simulink model "Supplementary"  (R2021a)
(part 22 of 44)

  | 59.9400000000000	0.0230096000000000	0	0.251530791000000	0.179781140000000	-0.315026171000000	-0.0424638370000000	0	0.0447050030000000	0.252430607000000	0.117599632000000	-0.0562562650000000	0	-0.250118815000000	0.495220037000000	0.448104106000000	0.0380873640000000	0	0.457102020000000	-0.0355396720000000	0.0629174220000000	0.0269596900000000	0	0.0225587780000000	-0.198933159000000	-0.173880731000000	0.0329760380000000	0	-0.0120823110000000	-0.612381407000000	-0.0657713680000000
  | 59.9500000000000	0.0225821490000000	0	0.251965335000000	0.182330207000000	-0.313827770000000	-0.0430235900000000	0	0.0421946840000000	0.257386793000000	0.122104378000000	-0.0556942900000000	0	-0.251945003000000	0.496017229000000	0.452844988000000	0.0383586100000000	0	0.457327004000000	-0.0375596220000000	0.0611753260000000	0.0272837990000000	0	0.0224268220000000	-0.204964025000000	-0.174486467000000	0.0318457760000000	0	-0.0143088790000000	-0.593791789000000	-0.0553758650000000
  | 59.9600000000000	0.0221491290000000	0	0.252374684000000	0.184928876000000	-0.312584084000000	-0.0435777230000000	0	0.0396661030000000	0.262350951000000	0.126656532000000	-0.0551323150000000	0	-0.253771190000000	0.496814420000000	0.457585870000000	0.0386330400000000	0	0.457550556000000	-0.0396389520000000	0.0594276930000000	0.0275966060000000	0	0.0222726010000000	-0.210808995000000	-0.174988248000000	0.0307155150000000	0	-0.0165354480000000	-0.575202171000000	-0.0449803630000000
  | 59.9700000000000	0.0217105950000000	0	0.252758657000000	0.187577226000000	-0.311294639000000	-0.0441262360000000	0	0.0371192600000000	0.267323082000000	0.131256095000000	-0.0545703400000000	0	-0.255597377000000	0.497611611000000	0.462326751000000	0.0389105420000000	0	0.457772456000000	-0.0417758020000000	0.0576755610000000	0.0278981090000000	0	0.0220961140000000	-0.216468068000000	-0.175386074000000	0.0295852530000000	0	-0.0187620170000000	-0.556612554000000	-0.0345848600000000
  | 59.9800000000000	0.0212666040000000	0	0.253117069000000	0.190275337000000	-0.309958962000000	-0.0446691290000000	0	0.0345541550000000	0.272303184000000	0.135903067000000	-0.0540083650000000	0	-0.257423565000000	0.498408802000000	0.467067633000000	0.0391910020000000	0	0.457992479000000	-0.0439683140000000	0.0559199710000000	0.0281883110000000	0	0.0218973610000000	-0.221941246000000	-0.175679945000000	0.0284549920000000	0	-0.0209885860000000	-0.538022936000000	-0.0241893580000000
  | 59.9900000000000	0.0208172120000000	0	0.253449740000000	0.193023290000000	-0.308576578000000	-0.0452064030000000	0	0.0319707890000000	0.277291258000000	0.140597448000000	-0.0534388670000000	0	-0.259237508000000	0.499147350000000	0.471723171000000	0.0394743080000000	0	0.458210403000000	-0.0462146270000000	0.0541619620000000	0.0284672090000000	0	0.0216763420000000	-0.227228527000000	-0.175869861000000	0.0272789170000000	0	-0.0232242500000000	-0.519210865000000	-0.0136702450000000
  | 60	0.0203624760000000	0	0.253756485000000	0.195821163000000	-0.307147013000000	-0.0457379070000000	0	0.0293694050000000	0.282286131000000	0.145337530000000	-0.0528242280000000	0	-0.260977987000000	0.499534036000000	0.475866645000000	0.0397603470000000	0	0.458426005000000	-0.0485128840000000	0.0524025740000000	0.0287338890000000	0	0.0214328760000000	-0.232325463000000	-0.175953350000000	0.0258279680000000	0	-0.0255144850000000	-0.499064078000000	-0.00240947200000000]
StopFcn:
  | clc
  | close all
  | 
  | T = Time.Data(:);
  | 
  | 
  | LeftThighF = LThighF.Data(:,:);
  | LeftThighT = LThighT.Data(:,:);
  | LeftThighS = LThighS.Data(:,:);
  | LeftKnee   = LKnee.Data(:,:);
  | LeftAnkle  = LAnkle.Data(:,:);
  | 
  | RightThighF = RThighF.Data(:,:);
  | RightThighT = RThighT.Data(:,:);
  | RightThighS = RThighS.Data(:,:);
  | RightKnee   = RKnee.Data(:,:);
  | RightAnkle  = RAnkle.Data(:,:);
  | 
  | 
  | LeftThighFtorque = LThighFtorque.Data(:);
  | LeftThighTtorque = LThighTtorque.Data(:);
  | LeftThighStorque = LThighStorque.Data(:);
  | LeftKneetorque   = LKneetorque.Data(:);
  | LeftAnkletorque  = LAnkletorque.Data(:);
  | 
  | RightThighFtorque = RThighFtorque.Data(:);
  | RightThighTtorque = RThighTtorque.Data(:);
  | RightThighStorque = RThighStorque.Data(:);
  | RightKneetorque   = RKneetorque.Data(:);
  | RightAnkletorque  = RAnkletorque.Data(:);
  | 
  | 
  | figure
  | subplot(4,2,2)
  | plot(T,RightThighF(:,1),'g',T,RightThighF(:,2),'b',T,RightThighF(:,3),'--m' ,'LineWidth',3)
  | legend({'\theta_{Ref}','\theta_{Simscape}','\theta_{Simulink}'}, 'Location','northeast', 'FontSize',10,'FontName', 'Times New Roman', 'FontWeight', 'bold')
  | xlabel('Time (Sec)', 'FontSize',10,'FontName', 'Times New Roman', 'FontWeight', 'bold' )
  | ylabel('Position (Degree)', 'FontSize',10,'FontName', 'Times New Roman', 'FontWeight', 'bold' )
  | title('Right Frontal Hip Position', 'FontSize',10,'FontName', 'Times New Roman' , 'FontWeight', 'bold')
  | ax = gca;
  | ax.FontSize = 10;
  | ax.FontName = 'Times New Roman';
  | ax.FontWeight = 'bold';
  | grid on
  | 
  | 
  | 
  | subplot(4,2,4)
  | plot(T,RightThighS(:,1),'g',T,RightThighS(:,2),'b',T,RightThighS(:,3),'--m' ,'LineWidth',3)
  | legend({'\theta_{Ref}','\theta_{Simscape}','\theta_{Simulink}'}, 'Location','northeast', 'FontSize',10,'FontName', 'Times New Roman', 'FontWeight', 'bold')
  | xlabel('Time (Sec)', 'FontSize',10,'FontName', 'Times New Roman', 'FontWeight', 'bold' )
  | ylabel('Position (Degree)', 'FontSize',10,'FontName', 'Times New Roman', 'FontWeight', 'bold' )
  | title('Right Saggital Hip Position', 'FontSize',10,'FontName', 'Times New Roman' , 'FontWeight', 'bold')
  | ax = gca;
  | ax.FontSize = 10;
  | ax.FontName = 'Times New Roman';
  | ax.FontWeight = 'bold';
  | grid on
  | 
  | 
  | 
  | subplot(4,2,6)
  | plot(T,RightKnee(:,1),'g',T,RightKnee(:,2),'b',T,RightKnee(:,3),'--m' ,'LineWidth',3)
  | legend({'\theta_{Ref}','\theta_{Simscape}','\theta_{Simulink}'}, 'Location','northeast', 'FontSize',10,'FontName', 'Times New Roman', 'FontWeight', 'bold')
  | xlabel('Time (Sec)', 'FontSize',10,'FontName', 'Times New Roman', 'FontWeight', 'bold' )
  | ylabel('Position (Degree)', 'FontSize',10,'FontName', 'Times New Roman', 'FontWeight', 'bold' )
  | title('Right Knee Position', 'FontSize',10,'FontName', 'Times New Roman' , 'FontWeight', 'bold')
  | ax = gca;
  | ax.FontSize = 10;
  | ax.FontName = 'Times New Roman';
  | ax.FontWeight = 'bold';
  | grid on
  | 
  | 
  | 
  | 
  | subplot(4,2,8)
  | plot(T,RightAnkle(:,1),'g',T,RightAnkle(:,2),'b',T,RightAnkle(:,3),'--m' ,'LineWidth',3)
  | legend({'\theta_{Ref}','\theta_{Simscape}','\theta_{Simulink}'}, 'Location','northeast', 'FontSize',10,'FontName', 'Times New Roman', 'FontWeight', 'bold')
  | xlabel('Time (Sec)', 'FontSize',10,'FontName', 'Times New Roman', 'FontWeight', 'bold' )
  | ylabel('Position (Degree)', 'FontSize',10,'FontName', 'Times New Roman', 'FontWeight', 'bold' )
  | title('Right Ankle Position', 'FontSize',10,'FontName', 'Times New Roman' , 'FontWeight', 'bold')
  | ax = gca;
  | ax.FontSize = 10;
  | ax.FontName = 'Times New Roman';
  | ax.FontWeight = 'bold';
  | grid on
  | 
  | 
  | subplot(4,2,1)
  | plot(T,LeftThighF(:,1),'g',T,LeftThighF(:,2),'b',T,LeftThighF(:,3),'--m' ,'LineWidth',3)
  | legend({'\theta_{Ref}','\theta_{Simscape}','\theta_{Simulink}'}, 'Location','northeast', 'FontSize',10,'FontName', 'Times New Roman', 'FontWeight', 'bold')
  | xlabel('Time (Sec)', 'FontSize',10,'FontName', 'Times New Roman', 'FontWeight', 'bold' )
  | ylabel('Position (Degree)', 'FontSize',10,'FontName', 'Times New Roman', 'FontWeight', 'bold' )
  | title('Left Frontal Hip Position', 'FontSize',10,'FontName', 'Times New Roman' , 'FontWeight', 'bold')
  | ax = gca;
  | ax.FontSize = 10;
  | ax.FontName = 'Times New Roman';
  | ax.FontWeight = 'bold';
  | grid on
  | 
  | 
  | 
  | subplot(4,2,3)
  | plot(T,LeftThighS(:,1),'g',T,LeftThighS(:,2),'b',T,LeftThighS(:,3),'--m' ,'LineWidth',3)
  | legend({'\theta_{Ref}','\theta_{Simscape}','\theta_{Simulink}'}, 'Location','northeast', 'FontSize',10,'FontName', 'Times New Roman', 'FontWeight', 'bold')
  | xlabel('Time (Sec)', 'FontSize',10,'FontName', 'Times New Roman', 'FontWeight', 'bold' )
  | ylabel('Position (Degree)', 'FontSize',10,'FontName', 'Times New Roman', 'FontWeight', 'bold' )
  | title('Left Saggital Hip Position', 'FontSize',10,'FontName', 'Times New Roman' , 'FontWeight', 'bold')
  | ax = gca;
  | ax.FontSize = 10;
  | ax.FontName = 'Times New Roman';
  | ax.FontWeight = 'bold';
  | grid on
  | 
  | 
  | subplot(4,2,5)
  | plot(T,LeftKnee(:,1),'g',T,LeftKnee(:,2),'b',T,LeftKnee(:,3),'--m' ,'LineWidth',3)
  | legend({'\theta_{Ref}','\theta_{Simscape}','\theta_{Simulink}'}, 'Location','northeast', 'FontSize',10,'FontName', 'Times New Roman', 'FontWeight', 'bold')
  | xlabel('Time (Sec)', 'FontSize',10,'FontName', 'Times New Roman', 'FontWeight', 'bold' )
  | ylabel('Position (Degree)', 'FontSize',10,'FontName', 'Times New Roman', 'FontWeight', 'bold' )
  | title('Left Knee Position', 'FontSize',10,'FontName', 'Times New Roman' , 'FontWeight', 'bold')
  | ax = gca;
  | ax.FontSize = 10;
  | ax.FontName = 'Times New Roman';
  | ax.FontWeight = 'bold';
  | grid on
  | 
  | 
  | subplot(4,2,7)
  | plot(T,LeftAnkle(:,1),'g',T,LeftAnkle(:,2),'b',T,LeftAnkle(:,3),'--m' ,'LineWidth',3)
  | legend({'\theta_{Ref}','\theta_{Simscape}','\theta_{Simulink}'}, 'Location','northeast', 'FontSize',10,'FontName', 'Times New Roman', 'FontWeight', 'bold')
  | xlabel('Time (Sec)', 'FontSize',10,'FontName', 'Times New Roman', 'FontWeight', 'bold' )
  | ylabel('Position (Degree)', 'FontSize',10,'FontName', 'Times New Roman', 'FontWeight', 'bold' )
  | title('Left Ankle Position', 'FontSize',10,'FontName', 'Times New Roman' , 'FontWeight', 'bold')
  | ax = gca;
  | ax.FontSize = 10;
  | ax.FontName = 'Times New Roman';
  | ax.FontWeight = 'bold';
  | grid on
  | 
  | 
  | figure
  | subplot 221
  | plot(T,RightThighFtorque,'b',T,LeftThighFtorque,'m' ,'LineWidth',3)
  | legend({'\tau_{Right}','\tau_{Left}'}, 'Location','northeast', 'FontSize',10,'FontName', 'Times New Roman', 'FontWeight', 'bold')
  | xlabel('Time (Sec)', 'FontSize',10,'FontName', 'Times New Roman', 'FontWeight', 'bold' )
  | ylabel('Torque (N.m)', 'FontSize',10,'FontName', 'Times New Roman', 'FontWeight', 'bold' )
  | title('Frontal Hip Torque', 'FontSize',10,'FontName', 'Times New Roman' , 'FontWeight', 'bold')
  | ax = gca;
  | ax.FontSize = 10;
  | ax.FontName = 'Times New Roman';
  | ax.FontWeight = 'bold';
  | grid on
  | 
  | 
  | 
  | 
  | subplot 222
  | plot(T,RightThighStorque,'b',T,LeftThighStorque,'m' ,'LineWidth',3)
  | legend({'\tau_{Right}','\tau_{Left}'}, 'Location','northeast', 'FontSize',10,'FontName', 'Times New Roman', 'FontWeight', 'bold')
  | xlabel('Time (Sec)', 'FontSize',10,'FontName', 'Times New Roman', 'FontWeight', 'bold' )
  | ylabel('Torque (N.m)', 'FontSize',10,'FontName', 'Times New Roman', 'FontWeight', 'bold' )
  | title('Saggital Hip Torque', 'FontSize',10,'FontName', 'Times New Roman' , 'FontWeight', 'bold')
  | ax = gca;
  | ax.FontSize = 10;
  | ax.FontName = 'Times New Roman';
  | ax.FontWeight = 'bold';
  | grid on
  | 
  | 
  | subplot 223
  | plot(T,RightKneetorque,'b',T,LeftKneetorque,'m' ,'LineWidth',3)
  | legend({'\tau_{Right}','\tau_{Left}'}, 'Location','northeast', 'FontSize',10,'FontName', 'Times New Roman', 'FontWeight', 'bold')
  | xlabel('Time (Sec)', 'FontSize',10,'FontName', 'Times New Roman', 'FontWeight', 'bold' )
  | ylabel('Torque (N.m)', 'FontSize',10,'FontName', 'Times New Roman', 'FontWeight', 'bold' )
  | title('Knee Torque', 'FontSize',10,'FontName', 'Times New Roman' , 'FontWeight', 'bold')
  | ax = gca;
  | ax.FontSize = 10;
  | ax.FontName = 'Times New Roman';
  | ax.FontWeight = 'bold';
  | grid on
  | 
  | 
  | subplot(2,2,4)
  | plot(T,RightAnkletorque,'b',T,LeftAnkletorque,'m' ,'LineWidth',3)
  | legend({'\tau_{Right}','\tau_{Left}'}, 'Location','northeast', 'FontSize',10,'FontName', 'Times New Roman', 'FontWeight', 'bold')
  | xlabel('Time (Sec)', 'FontSize',10,'FontName', 'Times New Roman', 'FontWeight', 'bold' )
  | ylabel('Torque (N.m)', 'FontSize',10,'FontName', 'Times New Roman', 'FontWeight', 'bold' )
  | title('Ankle Torque', 'FontSize',10,'FontName', 'Times New Roman' , 'FontWeight', 'bold')
  | ax = gca;
  | ax.FontSize = 10;
  | ax.FontName = 'Times New Roman';
  | ax.FontWeight = 'bold';
  | grid on
undefined symbols (not defined in the file): X, Y, Z
libraries: sm_lib x34, nesl_utility x21
settings Model: Creator=Mohammadhadi Sarajchi  LastModifiedBy=MS2209
settings DataIOCC: SaveOutput=off  SignalLogging=off  DSMLogging=off  SaveTime=off  ReturnWorkspaceOutputs=off

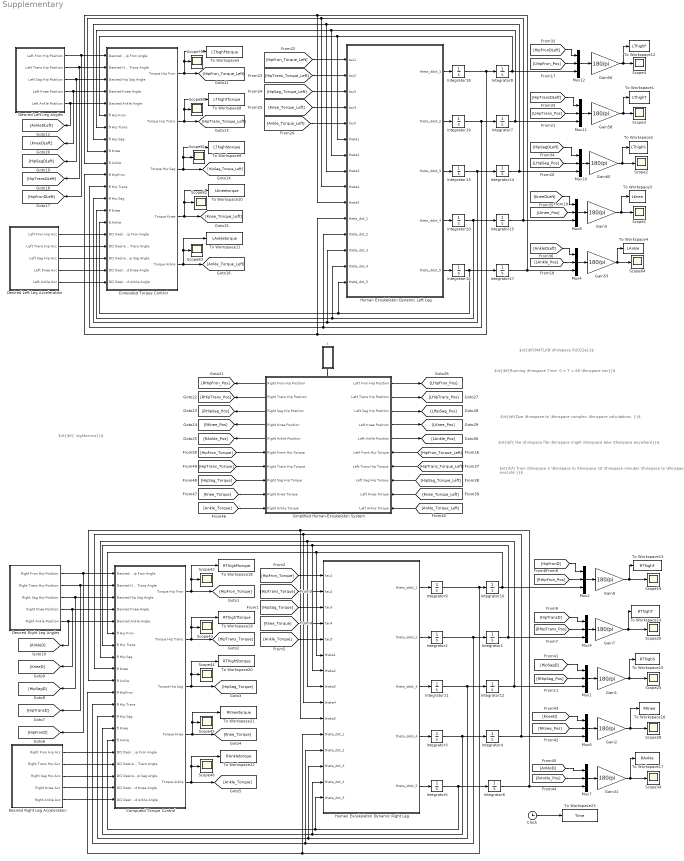
== system Supplementary ==
  note: $\it{\bf{MATLAB \thinspace R2021a}}$
  note: $\it{\bf{ \rightarrow}}$
  note: $\it{\bf{Running \thinspace Time: 0 < T < 60 \thinspace sec}}$
  note: $\it{\bf{ from \thinspace 5 \thinspace to \thinspace 10 \thinspace minutes \thinspace to \thinspace execute.}}$
  note: $\it{\bf{ the \thinspace file \thinspace might \thinspace take \thinspace anywhere}}$
  note: $\it{\bf{Due \thinspace to \thinspace complex \thinspace calculations, }}$
  Clock : Clock
  Computed Torque Control : Subsystem
      mask Display:
      | port_label('output',1,'\tau_{Hip FRon}','texmode','on');
      | port_label('output',2,'\tau_{Hip Trans}','texmode','on');
      | port_label('output',3,'\tau_{Hip Sag}','texmode','on');
      | port_label('output',4,'\tau_{Knee}','texmode','on');
      | port_label('output',5,'\tau_{Ankle}','texmode','on');
      | 
      | 
      | 
      | port_label('input',1,'\theta_d_{Hip Fron}','texmode','on');
      | port_label('input',2,'\theta_d_{Hip Trans}','texmode','on');
      | port_label('input',3,'\theta_d_{Hip Sag}','texmode','on');
      | port_label('input',4,'\theta_d_{ Knee}','texmode','on');
      | port_label('input',5,'\theta_d_{ Ankle}','texmode','on');
      | 
      | port_label('input',6,'\theta_{Hip Fron}','texmode','on');
      | port_label('input',7,'\theta_{Hip Trans}','texmode','on');
      | port_label('input',8,'\theta_{Hip Sag}','texmode','on');
      | port_label('input',9,'\theta_{Shank}','texmode','on');
      | port_label('input',10,'\theta_{Ankle}','texmode','on');
      | 
      | port_label('input',11,'\theta\prime_{Hip Fron}','texmode','on');
      | port_label('input',12,'\theta\prime_{Hip Trans}','texmode','on');
      | port_label('input',13,'\theta\prime_{Hip Sag}','texmode','on');
      | port_label('input',14,'\theta\prime_{Knee}','texmode','on');
      | port_label('input',15,'\theta\prime_{Ankle}','texmode','on');
      | 
      | port_label('input',16,'Ӫ_d_{ Hip Fron}','texmode','on');
      | port_label('input',17,'Ӫ_d_{ Hip Trans}','texmode','on');
      | port_label('input',18,'Ӫ_d_{ Hip Sag}','texmode','on');
      | port_label('input',19,'Ӫ_d_{ Knee}','texmode','on');
      | port_label('input',20,'Ӫ_d_{ Ankle}','texmode','on');
  "Computed Torque Control " : Subsystem
      mask Display:
      | port_label('output',1,'\tau_{Hip FRon}','texmode','on');
      | port_label('output',2,'\tau_{Hip Trans}','texmode','on');
      | port_label('output',3,'\tau_{Hip Sag}','texmode','on');
      | port_label('output',4,'\tau_{Knee}','texmode','on');
      | port_label('output',5,'\tau_{Ankle}','texmode','on');
      | 
      | 
      | 
      | port_label('input',1,'\theta_d_{Hip Fron}','texmode','on');
      | port_label('input',2,'\theta_d_{Hip Trans}','texmode','on');
      | port_label('input',3,'\theta_d_{Hip Sag}','texmode','on');
      | port_label('input',4,'\theta_d_{ Knee}','texmode','on');
      | port_label('input',5,'\theta_d_{ Ankle}','texmode','on');
      | 
      | port_label('input',6,'\theta_{Hip Fron}','texmode','on');
      | port_label('input',7,'\theta_{Hip Trans}','texmode','on');
      | port_label('input',8,'\theta_{Hip Sag}','texmode','on');
      | port_label('input',9,'\theta_{Shank}','texmode','on');
      | port_label('input',10,'\theta_{Ankle}','texmode','on');
      | 
      | port_label('input',11,'\theta\prime_{Hip Fron}','texmode','on');
      | port_label('input',12,'\theta\prime_{Hip Trans}','texmode','on');
      | port_label('input',13,'\theta\prime_{Hip Sag}','texmode','on');
      | port_label('input',14,'\theta\prime_{Knee}','texmode','on');
      | port_label('input',15,'\theta\prime_{Ankle}','texmode','on');
      | 
      | port_label('input',16,'Ӫ_d_{ Hip Fron}','texmode','on');
      | port_label('input',17,'Ӫ_d_{ Hip Trans}','texmode','on');
      | port_label('input',18,'Ӫ_d_{ Hip Sag}','texmode','on');
      | port_label('input',19,'Ӫ_d_{ Knee}','texmode','on');
      | port_label('input',20,'Ӫ_d_{ Ankle}','texmode','on');
  Desired Left Leg Acceleration : Subsystem
      mask Display:
      | port_label('output',1,'Ӫ_d_{ Hip Frontal}','texmode','on');
      | port_label('output',2,'Ӫ_d_{ Hip Trans}','texmode','on');
      | port_label('output',3,'Ӫ_d_{ Hip Saggital}','texmode','on');
      | port_label('output',4,'Ӫ_d_{ Knee}','texmode','on');
      | port_label('output',5,'Ӫ_d_{ Ankle}','texmode','on');
  Desired Left Leg Angles : Subsystem
      mask Display:
      | port_label('output',1,'\theta_d_{ Hip Frontal}','texmode','on');
      | port_label('output',2,'\theta_d_{ Hip Trans}','texmode','on');
      | port_label('output',3,'\theta_d_{ Hip Saggital}','texmode','on');
      | port_label('output',4,'\theta_d_{ Knee}','texmode','on');
      | port_label('output',5,'\theta_d_{ Ankle}','texmode','on');
  Desired Right Leg Acceleration : Subsystem
      mask Display:
      | port_label('output',1,'Ӫ_d_{ Hip Frontal}','texmode','on');
      | port_label('output',2,'Ӫ_d_{ Hip Trans}','texmode','on');
      | port_label('output',3,'Ӫ_d_{ Hip Saggital}','texmode','on');
      | port_label('output',4,'Ӫ_d_{ Knee}','texmode','on');
      | port_label('output',5,'Ӫ_d_{ Ankle}','texmode','on');
  Desired Right Leg Angles : Subsystem
      mask Display:
      | port_label('output',1,'\theta_d_{ Hip Frontal}','texmode','on');
      | port_label('output',2,'\theta_d_{ Hip Trans}','texmode','on');
      | port_label('output',3,'\theta_d_{ Hip Saggital}','texmode','on');
      | port_label('output',4,'\theta_d_{ Knee}','texmode','on');
      | port_label('output',5,'\theta_d_{ Ankle}','texmode','on');
  Gain{1..3,7,9,31,53,56,58,60} (10 alike) : Gain  Gain=180/pi
  Human Exoskeleton Dynamic Right Leg : MATLAB Function  TreatAsAtomicUnit=on
  Human Exoskeleton Dynamic Left Leg : MATLAB Function  TreatAsAtomicUnit=on
  I : Subsystem
  Integrator{1..11,13,15..20} (18 alike) : Integrator
  Integrator12 : Integrator  InitialCondition=pi/2*0
  Integrator14 : Integrator  InitialCondition=pi/2*0
  Mux{1..2,4,6..12} (10 alike) : Mux  Inputs=3
  Scope{1..4,19..20,25,28,34,42..46,64,79..83} (20 alike) : Scope
  Simplified Human-Exoskeleton System : Subsystem
      settings: PortSchema="{\"entries\":[{\"content\":{\"sides\":[{\"content\":{\"connectorIds\":[\"Out6\",\"Out7\",\"Out8\",\"Out9\",\"Out10\",\"In1\",\"In2\",\"In3\",\"In4\",\"In5\"]},\"type\":\"ConnectorPlacement.EquallySpacedRectSide\",\"uuid\":\"44bd4c95-62cb-4344-b9a9-b6829513d594\"},{\"content\":{\"connectorIds\":[\"Out1\",\"Out2\",\"Out3\",\"Out4\",\"Out5\",\"In6\",\"In7\",\"In8\",\"In9\",\"In10\"],\"side\":\"RIGHT\"},\"type\":\"ConnectorPlacement.EquallySpacedRectSide\",\"uuid\":\"7479bc40-820f-47da-a6f3-d0e40a2d4702\"},{\"content\":{\"connectorIds\":[\"LConn1\"],\"side\":\"TOP\"},\"type\":\"ConnectorPlacement.EquallySpacedRectSide\",\"uuid\":\"52723317-f3a9-47a3-98e1-7d76bcec4505\"}]},\"type\":\"ConnectorPlacement.EquallySpacedConnector\",\"uuid\":\"54affe45-471d-4584-a1b2-79c80a401fa7\"}],\"packageUris\":[\"http://schema.mathworks.com/mf0/Connector/R2020b\"],\"version\":\"1.0\"}"
  To Workspace1 : ToWorkspace  VariableName=LThighT  SaveFormat=Timeseries  SampleTime=-1
  To Workspace10 : ToWorkspace  VariableName=LKneetorque  SaveFormat=Timeseries  SampleTime=-1
  To Workspace11 : ToWorkspace  VariableName=LAnkletorque  SaveFormat=Timeseries  SampleTime=-1
  To Workspace12 : ToWorkspace  VariableName=LThighF  SaveFormat=Timeseries  SampleTime=-1
  To Workspace13 : ToWorkspace  VariableName=RThighF  SaveFormat=Timeseries  SampleTime=-1
  To Workspace14 : ToWorkspace  VariableName=RThighT  SaveFormat=Timeseries  SampleTime=-1
  To Workspace15 : ToWorkspace  VariableName=RThighS  SaveFormat=Timeseries  SampleTime=-1
  To Workspace16 : ToWorkspace  VariableName=RKnee  SaveFormat=Timeseries  SampleTime=-1
  To Workspace17 : ToWorkspace  VariableName=RAnkle  SaveFormat=Timeseries  SampleTime=-1
  To Workspace18 : ToWorkspace  VariableName=RThighFtorque  SaveFormat=Timeseries  SampleTime=-1
  To Workspace19 : ToWorkspace  VariableName=RThighTtorque  SaveFormat=Timeseries  SampleTime=-1
  To Workspace2 : ToWorkspace  VariableName=LThighS  SaveFormat=Timeseries  SampleTime=-1
  To Workspace20 : ToWorkspace  VariableName=RThighStorque  SaveFormat=Timeseries  SampleTime=-1
  To Workspace21 : ToWorkspace  VariableName=RKneetorque  SaveFormat=Timeseries  SampleTime=-1
  To Workspace22 : ToWorkspace  VariableName=RAnkletorque  SaveFormat=Timeseries  SampleTime=-1
  To Workspace23 : ToWorkspace  VariableName=Time  SaveFormat=Timeseries  SampleTime=-1
  To Workspace3 : ToWorkspace  VariableName=LKnee  SaveFormat=Timeseries  SampleTime=-1
  To Workspace4 : ToWorkspace  VariableName=LAnkle  SaveFormat=Timeseries  SampleTime=-1
  To Workspace5 : ToWorkspace  VariableName=LThighFtorque  SaveFormat=Timeseries  SampleTime=-1
  To Workspace8 : ToWorkspace  VariableName=LThighTtorque  SaveFormat=Timeseries  SampleTime=-1
  To Workspace9 : ToWorkspace  VariableName=LThighStorque  SaveFormat=Timeseries  SampleTime=-1
  wires:
  Desired Right Leg Acceleration/3(Right Sag Hip Acc) -> Computed Torque Control/18(DD Desired Hip Sag Angle)
  Computed Torque Control/5(Torque Ankle) -> To Workspace22/1, Scope46/1, [Ankle_Torque]
  Integrator4/1 -> Computed Torque Control/9(θ Knee), Human Exoskeleton Dynamic Right Leg/9(theta4), Mux6/3
  Integrator3/1 -> Integrator4/1, Computed Torque Control/14(θ́ Knee), Human Exoskeleton Dynamic Right Leg/14(theta_dot_4)
  Integrator6/1 -> Computed Torque Control/10(θ Ankle), Human Exoskeleton Dynamic Right Leg/10(theta5), Mux7/3
  Desired Right Leg Acceleration/4(Right Knee Acc) -> Computed Torque Control/19(DD Desired Knee Angle)
  Computed Torque Control/3(Torque Hip Sag) -> To Workspace20/1, Scope44/1, [HipSag_Torque]
  Integrator1/1 -> Mux9/3, Computed Torque Control/7(θ Hip Trans), Human Exoskeleton Dynamic Right Leg/7(theta2)
  Desired Right Leg Acceleration/1(Right Fron Hip Acc) -> Computed Torque Control/16(DD Desired Hip Fron Angle)
  Computed Torque Control/1(Torque Hip Fron) -> To Workspace18/1, Scope42/1, [HipFron_Torque]
  Computed Torque Control/4(Torque Knee) -> To Workspace21/1, Scope45/1, [Knee_Torque]
  Computed Torque Control/2(Torque Hip Trans) -> To Workspace19/1, Scope43/1, [HipTrans_Torque]
  Integrator5/1 -> Integrator6/1, Computed Torque Control/15(θ́ Ankle), Human Exoskeleton Dynamic Right Leg/15(theta_dot_5)
  Desired Right Leg Acceleration/5(Right Ankle Acc) -> Computed Torque Control/20(DD Desired Ankle Angle)
  [Knee_Torque] -> Human Exoskeleton Dynamic Right Leg/4(tau4)
  Human Exoskeleton Dynamic Right Leg/1(theta_ddot_1) -> Integrator9/1
  Human Exoskeleton Dynamic Right Leg/2(theta_ddot_2) -> Integrator2/1
  [HipSag_Torque] -> Human Exoskeleton Dynamic Right Leg/3(tau3)
  [HipFron_Torque] -> Human Exoskeleton Dynamic Right Leg/1(tau1)
  [HipTrans_Torque] -> Human Exoskeleton Dynamic Right Leg/2(tau2)
  [Ankle_Torque] -> Human Exoskeleton Dynamic Right Leg/5(tau5)
  Human Exoskeleton Dynamic Right Leg/3(theta_ddot_3) -> Integrator11/1
  Human Exoskeleton Dynamic Right Leg/5(theta_ddot_5) -> Integrator5/1
  Mux2/1 -> Gain9/1
  Human Exoskeleton Dynamic Right Leg/4(theta_ddot_4) -> Integrator3/1
  Integrator9/1 -> Integrator10/1, Computed Torque Control/11(θ́ HipFron), Human Exoskeleton Dynamic Right Leg/11(theta_dot_1)
  Integrator12/1 -> Mux1/3, Computed Torque Control/8(θ Hip Sag), Human Exoskeleton Dynamic Right Leg/8(theta3)
  Integrator10/1 -> Mux2/3, Computed Torque Control/6(θ Hip Fron), Human Exoskeleton Dynamic Right Leg/6(theta1)
  Integrator2/1 -> Integrator1/1, Computed Torque Control/12(θ́ Hip Trans), Human Exoskeleton Dynamic Right Leg/12(theta_dot_2)
  Desired Right Leg Acceleration/2(Right Trans Hip Acc) -> Computed Torque Control/17(DD Desired Hip Trans Angle)
  Integrator11/1 -> Integrator12/1, Computed Torque Control/13(θ́ Hip Sag), Human Exoskeleton Dynamic Right Leg/13(theta_dot_3)
  Clock/1 -> To Workspace23/1
  [Ankle_Torque_Left] -> Human Exoskeleton Dynamic Left Leg/5(tau5)
  Integrator13/1 -> Integrator14/1, Human Exoskeleton Dynamic Left Leg/13(theta_dot_3), "Computed Torque Control "/13(θ́ Hip Sag)
  Integrator16/1 -> Integrator17/1, Human Exoskeleton Dynamic Left Leg/15(theta_dot_5), "Computed Torque Control "/15(θ́ Ankle)
  Integrator15/1 -> Mux8/3, Human Exoskeleton Dynamic Left Leg/9(theta4), "Computed Torque Control "/9(θ Knee)
  Integrator14/1 -> Mux10/3, "Computed Torque Control "/8(θ Hip Sag), Human Exoskeleton Dynamic Left Leg/8(theta3)
  "Computed Torque Control "/4(Torque Knee) -> [Knee_Torque_Left], To Workspace10/1, Scope82/1
  Integrator7/1 -> Mux11/3, "Computed Torque Control "/7(θ Hip Trans), Human Exoskeleton Dynamic Left Leg/7(theta2)
  Integrator8/1 -> Mux12/3, "Computed Torque Control "/6(θ Hip Fron), Human Exoskeleton Dynamic Left Leg/6(theta1)
  "Computed Torque Control "/1(Torque Hip Fron) -> [HipFron_Torque_Left], To Workspace5/1, Scope79/1
  "Computed Torque Control "/5(Torque Ankle) -> [Ankle_Torque_Left], To Workspace11/1, Scope83/1
  [HipTrans_Torque_Left] -> Human Exoskeleton Dynamic Left Leg/2(tau2)
  Desired Left Leg Acceleration/2(Left Trans Hip Acc) -> "Computed Torque Control "/17(DD Desired Hip Trans Angle)
  Desired Left Leg Acceleration/1(Left Fron Hip Acc) -> "Computed Torque Control "/16(DD Desired Hip Fron Angle)
  Integrator19/1 -> Integrator7/1, Human Exoskeleton Dynamic Left Leg/12(theta_dot_2), "Computed Torque Control "/12(θ́ Hip Trans)
  Human Exoskeleton Dynamic Left Leg/2(theta_ddot_2) -> Integrator19/1
  Desired Left Leg Acceleration/5(Left Ankle Acc) -> "Computed Torque Control "/20(DD Desired Ankle Angle)
  Integrator20/1 -> Integrator15/1, Human Exoskeleton Dynamic Left Leg/14(theta_dot_4), "Computed Torque Control "/14(θ́ Knee)
  [HipFron_Torque_Left] -> Human Exoskeleton Dynamic Left Leg/1(tau1)
  Desired Left Leg Angles/5(Left Ankle Position) -> "Computed Torque Control "/5(Desired Ankle Angle), [AnkleDLeft]
  Desired Left Leg Acceleration/3(Left Sag Hip Acc) -> "Computed Torque Control "/18(DD Desired Hip Sag Angle)
  Desired Left Leg Angles/1(Left Fron Hip Position) -> "Computed Torque Control "/1(Desired Hip Fron Angle), [HipFronDLeft]
  "Computed Torque Control "/2(Torque Hip Trans) -> [HipTrans_Torque_Left], To Workspace8/1, Scope80/1
  Desired Left Leg Acceleration/4(Left Knee Acc) -> "Computed Torque Control "/19(DD Desired Knee Angle)
  Desired Left Leg Angles/2(Left Trans Hip Position) -> "Computed Torque Control "/2(Desired Hip Trans Angle), [HipTransDLeft]
  Human Exoskeleton Dynamic Left Leg/4(theta_ddot_4) -> Integrator20/1
  Human Exoskeleton Dynamic Left Leg/3(theta_ddot_3) -> Integrator13/1
  Integrator18/1 -> Integrator8/1, "Computed Torque Control "/11(θ́ HipFron), Human Exoskeleton Dynamic Left Leg/11(theta_dot_1)
  "Computed Torque Control "/3(Torque Hip Sag) -> [HipSag_Torque_Left], To Workspace9/1, Scope81/1
  Human Exoskeleton Dynamic Left Leg/1(theta_ddot_1) -> Integrator18/1
  Desired Left Leg Angles/3(Left Sag Hip Position) -> "Computed Torque Control "/3(Desired Hip Sag Angle), [HipSagDLeft]
  Human Exoskeleton Dynamic Left Leg/5(theta_ddot_5) -> Integrator16/1
  Desired Left Leg Angles/4(Left Knee Position) -> "Computed Torque Control "/4(Desired Knee Angle), [KneeDLeft]
  [Knee_Torque_Left] -> Human Exoskeleton Dynamic Left Leg/4(tau4)
  [HipSag_Torque_Left] -> Human Exoskeleton Dynamic Left Leg/3(tau3)
  Integrator17/1 -> "Computed Torque Control "/10(θ Ankle), Human Exoskeleton Dynamic Left Leg/10(theta5), Mux4/3
  [HipFron_Torque] -> Simplified Human-Exoskeleton System/1(Right Front Hip Torque)
  [HipTrans_Torque] -> Simplified Human-Exoskeleton System/2(Right Trans Hip Torque)
  [HipSag_Torque] -> Simplified Human-Exoskeleton System/3(Right Sag Hip Torque)
  [Knee_Torque] -> Simplified Human-Exoskeleton System/4(Right Knee Torque)
  [Ankle_Torque] -> Simplified Human-Exoskeleton System/5(Right Ankle Torque)
  [HipFron_Torque_Left] -> Simplified Human-Exoskeleton System/6(Left Front Hip Torque)
  [HipTrans_Torque_Left] -> Simplified Human-Exoskeleton System/7(Left Trans Hip Torque)
  [HipSag_Torque_Left] -> Simplified Human-Exoskeleton System/8(Left Sag Hip Torque)
  [Knee_Torque_Left] -> Simplified Human-Exoskeleton System/9(Left Knee Torque)
  [Ankle_Torque_Left] -> Simplified Human-Exoskeleton System/10(Left Ankle Torque)
  Desired Right Leg Angles/5(Right Ankle Position) -> Computed Torque Control/5(Desired Ankle Angle), [AnkleD]
  Desired Right Leg Angles/4(Right Knee Position) -> Computed Torque Control/4(Desired Knee Angle), [KneeD]
  Desired Right Leg Angles/3(Right Sag Hip Position) -> Computed Torque Control/3(Desired Hip Sag Angle), [HipSagD]
  Desired Right Leg Angles/2(Right Trans Hip Position) -> Computed Torque Control/2(Desired Hip Trans Angle), [HipTransD]
  Desired Right Leg Angles/1(Right Fron Hip Position) -> Computed Torque Control/1(Desired Hip Fron Angle), [HipFronD]
  [RHipFron_Pos] -> Mux2/2
  [RHipTrans_Pos] -> Mux9/2
  [HipFronD] -> Mux2/1
  Gain9/1 -> Scope19/1, To Workspace13/1
  Mux9/1 -> Gain7/1
  Gain7/1 -> To Workspace14/1, Scope20/1
  [HipTransD] -> Mux9/1
  Mux1/1 -> Gain1/1
  Gain1/1 -> To Workspace15/1, Scope25/1
  [RHipSag_Pos] -> Mux1/2
  [HipSagD] -> Mux1/1
  Mux6/1 -> Gain2/1
  Gain2/1 -> To Workspace16/1, Scope28/1
  [RKnee_Pos] -> Mux6/2
  [KneeD] -> Mux6/1
  Gain31/1 -> Scope34/1, To Workspace17/1
  Mux7/1 -> Gain31/1
  [RAnkle_Pos] -> Mux7/2
  [AnkleD] -> Mux7/1
  Mux4/1 -> Gain53/1
  Gain53/1 -> To Workspace4/1, Scope64/1
  [AnkleDLeft] -> Mux4/1
  [KneeDLeft] -> Mux8/1
  Mux8/1 -> Gain3/1
  Gain3/1 -> To Workspace3/1, Scope1/1
  [LAnkle_Pos] -> Mux4/2
  [LKnee_Pos] -> Mux8/2
  Mux10/1 -> Gain60/1
  [HipSagDLeft] -> Mux10/1
  Gain60/1 -> To Workspace2/1, Scope2/1
  Mux11/1 -> Gain58/1
  [HipTransDLeft] -> Mux11/1
  Gain58/1 -> Scope3/1, To Workspace1/1
  [LHipSag_Pos] -> Mux10/2
  [LHipTrans_Pos] -> Mux11/2
  Mux12/1 -> Gain56/1
  Gain56/1 -> To Workspace12/1, Scope4/1
  [LHipFron_Pos] -> Mux12/2
  [HipFronDLeft] -> Mux12/1
  Simplified Human-Exoskeleton System/5(Left Ankle Position) -> [LAnkle_Pos]
  Simplified Human-Exoskeleton System/4(Left Knee Position) -> [LKnee_Pos]
  Simplified Human-Exoskeleton System/3(Left Sag Hip Position) -> [LHipSag_Pos]
  Simplified Human-Exoskeleton System/2(Left Trans Hip Position) -> [LHipTrans_Pos]
  Simplified Human-Exoskeleton System/1(Left Fron Hip Position) -> [LHipFron_Pos]
  Simplified Human-Exoskeleton System/10(Right Ankle Position) -> [RAnkle_Pos]
  Simplified Human-Exoskeleton System/9(Right Knee Position) -> [RKnee_Pos]
  Simplified Human-Exoskeleton System/8(Right Sag Hip Position) -> [RHipSag_Pos]
  Simplified Human-Exoskeleton System/7(Right Trans Hip Position) -> [RHipTrans_Pos]
  Simplified Human-Exoskeleton System/6(Right Fron Hip Position) -> [RHipFron_Pos]
  connections:
  I/RConn1 -- Simplified Human-Exoskeleton System/LConn1
